simulink model "copy_final"  (R2013a)
settings: Solver=ode45  StartTime=0.0  StopTime=150  RelTol=1e-3
model workspace (MAT data in the model file):
  i = 2
undefined symbols (not defined in the file): sigbuilder_block
(part 1 of 3)
settings Model: Creator=User  LastModifiedBy=User
settings DebuggingCC: SolverPrmCheckMsg=none

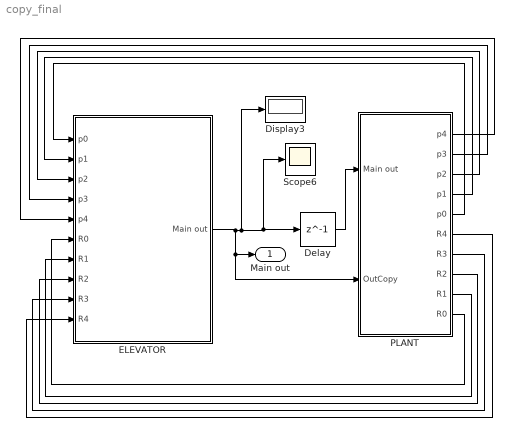
== system copy_final ==
  Delay : Delay  DelayLength=1  InitialCondition=0  SampleTime=1
  Display3 : Display
  ELEVATOR : Subsystem
  PLANT : Subsystem
  Scope6 : Scope
  Main out : Outport  OutDataTypeStr=int32
  wires:
  ELEVATOR/1(Main out) -> Scope6/1, Delay/1, Display3/1, PLANT/2(OutCopy), Main out/1
  Delay/1 -> PLANT/1(Main out)
  PLANT/5(p0) -> ELEVATOR/1(p0)
  PLANT/4("p1 ") -> ELEVATOR/2(p1)
  PLANT/3("p2 ") -> ELEVATOR/3(p2)
  PLANT/2("p3 ") -> ELEVATOR/4(p3)
  PLANT/1("p4 ") -> ELEVATOR/5(p4)
  PLANT/10(R0) -> ELEVATOR/6(R0)
  PLANT/9(R1) -> ELEVATOR/7(R1)
  PLANT/8(R2) -> ELEVATOR/8(R2)
  PLANT/7(R3) -> ELEVATOR/9(R3)
  PLANT/6(R4) -> ELEVATOR/10(R4)

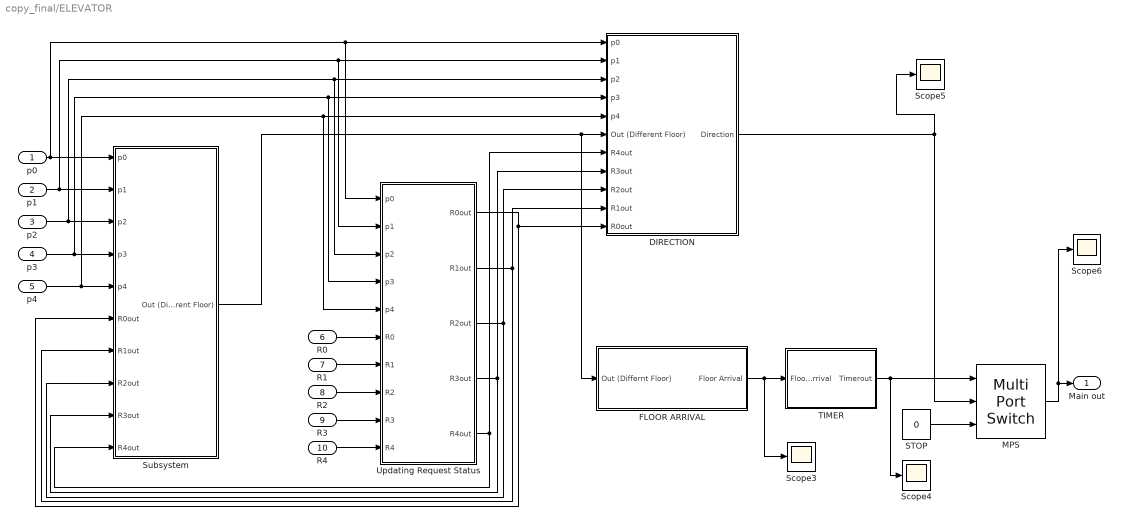
== system copy_final/ELEVATOR ==
  p0 : Inport  OutDataTypeStr=boolean
  p1 : Inport  Port=2  OutDataTypeStr=boolean
  p2 : Inport  Port=3  OutDataTypeStr=boolean
  p3 : Inport  Port=4  OutDataTypeStr=boolean
  p4 : Inport  Port=5  OutDataTypeStr=boolean  SampleTime=1
  R0 : Inport  Port=6  OutDataTypeStr=boolean
  R1 : Inport  Port=7  OutDataTypeStr=boolean
  R2 : Inport  Port=8  OutDataTypeStr=boolean
  R3 : Inport  Port=9  OutDataTypeStr=boolean
  R4 : Inport  Port=10  OutDataTypeStr=boolean
  DIRECTION : Subsystem
  FLOOR ARRIVAL : Subsystem
  "MPS " : MultiPortSwitch  DataPortOrder=Zero-based contiguous  Inputs=2  DiagnosticForDefault=None  OutDataTypeStr=int32  InputSameDT=on
  STOP : Constant  Value=0  OutDataTypeStr=int32
  Scope{3..6} (4 alike) : Scope
      Scope3 settings: SaveName=ScopeData76
      Scope4 settings: SaveName=ScopeData78
      Scope5 settings: SaveName=ScopeData8
      Scope6 settings: SaveName=ScopeData73
  Subsystem : Subsystem
  TIMER : Subsystem
  Updating Request Status : Subsystem
  Main out : Outport  OutDataTypeStr=int32
  wires:
  "MPS "/1 -> Scope6/1, Main out/1
  DIRECTION/1(" Direction ") -> "MPS "/2, Scope5/1
  TIMER/1(Timerout) -> "MPS "/1, Scope4/1
  FLOOR ARRIVAL/1(Floor Arrival) -> TIMER/1(Floor Arrival), Scope3/1
  p1/1 -> Updating Request Status/2(p1), DIRECTION/2(p1), Subsystem/2(p1)
  p2/1 -> Updating Request Status/3(p2), DIRECTION/3(p2), Subsystem/3(p2)
  p3/1 -> Updating Request Status/4(p3), DIRECTION/4(p3), Subsystem/4(p3)
  p4/1 -> Updating Request Status/5(p4), DIRECTION/5(p4), Subsystem/5(p4)
  Subsystem/1(Out (Different Floor)) -> FLOOR ARRIVAL/1(Out (Differnt Floor)), DIRECTION/6(Out (Different Floor))
  STOP/1 -> "MPS "/3
  Updating Request Status/1(R0out) -> Subsystem/6(R0out), DIRECTION/11(R0out)
  Updating Request Status/2(R1out) -> Subsystem/7(R1out), DIRECTION/10(R1out)
  Updating Request Status/3(R2out) -> Subsystem/8(R2out), DIRECTION/9(R2out)
  Updating Request Status/4(R3out) -> Subsystem/9(R3out), DIRECTION/8(R3out)
  Updating Request Status/5(R4out) -> Subsystem/10(R4out), DIRECTION/7(R4out)
  R1/1 -> Updating Request Status/7(R1)
  R2/1 -> Updating Request Status/8(R2)
  R3/1 -> Updating Request Status/9(R3)
  R4/1 -> Updating Request Status/10(R4)
  R0/1 -> Updating Request Status/6(R0)
  p0/1 -> DIRECTION/1(p0), Updating Request Status/1(p0), Subsystem/1(p0)

== system copy_final/PLANT ==
  Main out : Inport  OutDataTypeStr=int32
  OutCopy : Inport  Port=2  OutDataTypeStr=int32
  Calculating Position : Subsystem
  Live Request : Subsystem
  Position Id : Subsystem
  "p4 " : Outport  OutDataTypeStr=boolean
  "p3 " : Outport  Port=2  OutDataTypeStr=boolean
  "p2 " : Outport  Port=3  OutDataTypeStr=boolean
  "p1 " : Outport  Port=4  OutDataTypeStr=boolean
  p0 : Outport  Port=5  OutDataTypeStr=boolean
  R4 : Outport  Port=6  OutDataTypeStr=boolean
  R3 : Outport  Port=7  OutDataTypeStr=boolean
  R2 : Outport  Port=8  OutDataTypeStr=boolean
  R1 : Outport  Port=9  OutDataTypeStr=boolean
  R0 : Outport  Port=10  OutDataTypeStr=boolean
  wires:
  Live Request/1(R4) -> R4/1
  Live Request/2(R3) -> R3/1
  Live Request/3(R2) -> R2/1
  Live Request/4(R1) -> R1/1
  Live Request/5(R0) -> R0/1
  Position Id/1("p4 ") -> "p4 "/1
  Position Id/2("p3 ") -> "p3 "/1
  Position Id/3("p2 ") -> "p2 "/1
  Position Id/4("p1 ") -> "p1 "/1
  Position Id/5(p0) -> p0/1
  Calculating Position/1(position) -> Position Id/1(position)
  Main out/1 -> Calculating Position/1(Main out)
  OutCopy/1 -> Live Request/1(OutCopy)

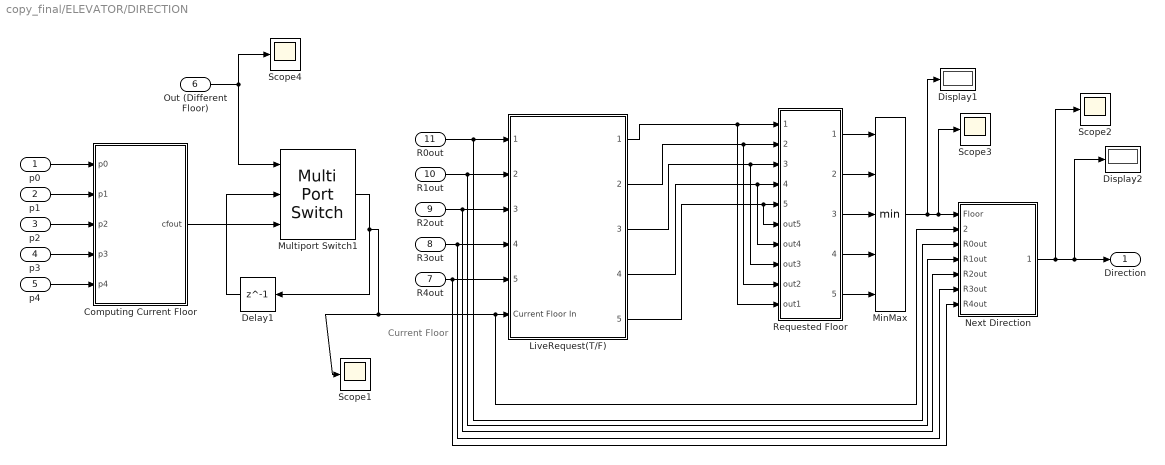
== system copy_final/ELEVATOR/DIRECTION ==
  note: Current Floor
  p0 : Inport  OutDataTypeStr=boolean
  p1 : Inport  Port=2  OutDataTypeStr=boolean
  p2 : Inport  Port=3  OutDataTypeStr=boolean
  p3 : Inport  Port=4  OutDataTypeStr=boolean
  p4 : Inport  Port=5  OutDataTypeStr=boolean
  Out (Different Floor) : Inport  Port=6  OutDataTypeStr=boolean
  R4out : Inport  Port=7  OutDataTypeStr=boolean
  R3out : Inport  Port=8  OutDataTypeStr=boolean
  R2out : Inport  Port=9  OutDataTypeStr=boolean
  R1out : Inport  Port=10  OutDataTypeStr=boolean
  R0out : Inport  Port=11  OutDataTypeStr=boolean
  "Computing Current Floor " : Subsystem
  Delay1 : Delay  DelayLength=1  SampleTime=1
  Display1 : Display
  Display2 : Display
  LiveRequest(T/F) : Subsystem
  MinMax : MinMax  Inputs=5  OutDataTypeStr=int32
  Multiport Switch1 : MultiPortSwitch  DataPortOrder=Zero-based contiguous  Inputs=2  DiagnosticForDefault=None  OutDataTypeStr=int32  InputSameDT=on
  Next Direction : Subsystem
  Requested Floor : Subsystem
  Scope{1..4} (4 alike) : Scope
      Scope1 settings: SaveName=ScopeData83
      Scope2 settings: SaveName=ScopeData47
      Scope3 settings: SaveName=ScopeData53
      Scope4 settings: SaveName=ScopeData84
  " Direction " : Outport  OutDataTypeStr=int32
  wires:
  p2/1 -> "Computing Current Floor "/3(p2)
  p3/1 -> "Computing Current Floor "/4(p3)
  p4/1 -> "Computing Current Floor "/5(p4)
  LiveRequest(T/F)/5 -> Requested Floor/6(out5), Requested Floor/5
  LiveRequest(T/F)/4 -> Requested Floor/4, Requested Floor/7(out4)
  Requested Floor/1(F0Out) -> MinMax/1
  Requested Floor/2(F1Out) -> MinMax/2
  Requested Floor/3(F2Out) -> MinMax/3
  Requested Floor/4(F3Out) -> MinMax/4
  Requested Floor/5(F4Out) -> MinMax/5
  p0/1 -> "Computing Current Floor "/1(p0)
  LiveRequest(T/F)/3 -> Requested Floor/8(out3), Requested Floor/3
  LiveRequest(T/F)/2 -> Requested Floor/9(out2), Requested Floor/2
  LiveRequest(T/F)/1 -> Requested Floor/10(out1), Requested Floor/1
  Next Direction/1(Direction) -> Scope2/1, Display2/1, " Direction "/1
  Multiport Switch1/1 -> Next Direction/2(Current Floor), LiveRequest(T/F)/6(Current Floor In), Scope1/1, Delay1/1
  MinMax/1 -> Next Direction/1(Floor), Scope3/1, Display1/1
  Out (Different Floor)/1 -> Scope4/1, Multiport Switch1/1
  p1/1 -> "Computing Current Floor "/2(p1)
  "Computing Current Floor "/1(cfout) -> Multiport Switch1/3
  Delay1/1 -> Multiport Switch1/2
  R1out/1 -> LiveRequest(T/F)/2, Next Direction/4(R1out)
  R2out/1 -> LiveRequest(T/F)/3, Next Direction/5(R2out)
  R3out/1 -> LiveRequest(T/F)/4, Next Direction/6(R3out)
  R4out/1 -> LiveRequest(T/F)/5, Next Direction/7(R4out)
  R0out/1 -> LiveRequest(T/F)/1, Next Direction/3(R0out)

== system copy_final/ELEVATOR/FLOOR ARRIVAL ==
  Out (Differnt Floor) : Inport  OutDataTypeStr=boolean
  " 1" : Logic  Operator=NOT  AllPortsSameDT=off  OutDataTypeStr=boolean
  Delay1 : Delay  DelayLength=1  SampleTime=1
  "Relational Operator " : Logic  AllPortsSameDT=off  OutDataTypeStr=boolean
  Scope{1..4} (4 alike) : Scope
      Scope1 settings: SaveName=ScopeData31
      Scope2 settings: SaveName=ScopeData32
      Scope3 settings: SaveName=ScopeData75
      Scope4 settings: SaveName=ScopeData77
  Floor Arrival : Outport  OutDataTypeStr=boolean
  wires:
  Out (Differnt Floor)/1 -> Scope1/1, Delay1/1, "Relational Operator "/1
  Delay1/1 -> Scope3/1, " 1"/1
  "Relational Operator "/1 -> Floor Arrival/1, Scope2/1
  " 1"/1 -> "Relational Operator "/2, Scope4/1

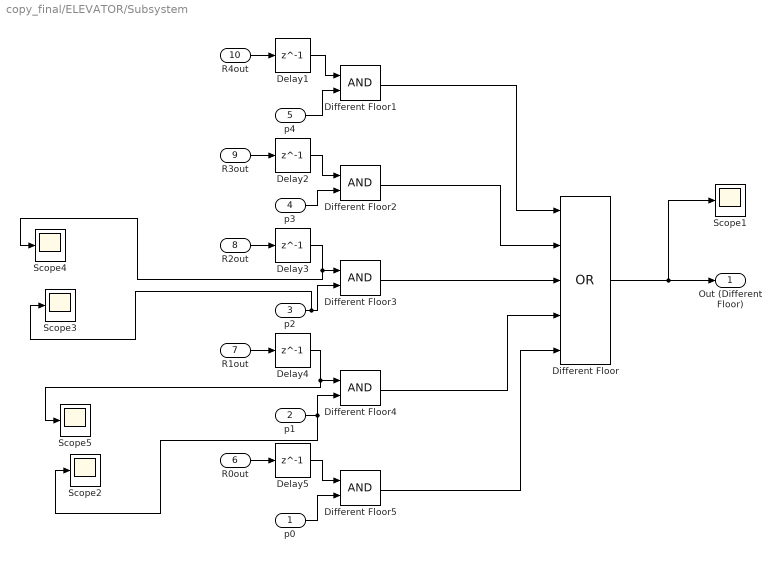
== system copy_final/ELEVATOR/Subsystem ==
  p0 : Inport  OutDataTypeStr=boolean
  p1 : Inport  Port=2  OutDataTypeStr=boolean
  p2 : Inport  Port=3  OutDataTypeStr=boolean
  p3 : Inport  Port=4  OutDataTypeStr=boolean
  p4 : Inport  Port=5  OutDataTypeStr=boolean  SampleTime=1
  R0out : Inport  Port=6  OutDataTypeStr=boolean
  R1out : Inport  Port=7  OutDataTypeStr=boolean
  R2out : Inport  Port=8  OutDataTypeStr=boolean
  R3out : Inport  Port=9  OutDataTypeStr=boolean
  R4out : Inport  Port=10  OutDataTypeStr=boolean
  Delay{1..5} (5 alike) : Delay  DelayLength=1  SampleTime=1
  Different Floor : Logic  Operator=OR  Inputs=5  AllPortsSameDT=off  OutDataTypeStr=boolean
  Different Floor{1..5} (5 alike) : Logic  AllPortsSameDT=off  OutDataTypeStr=boolean
  Scope{1..5} (5 alike) : Scope
      Scope1 settings: SaveName=ScopeData45
      Scope2 settings: SaveName=ScopeData46
      Scope3 settings: SaveName=ScopeData65
      Scope4 settings: SaveName=ScopeData66
      Scope5 settings: SaveName=ScopeData44
  Out (Different Floor) : Outport  OutDataTypeStr=boolean
  wires:
  R4out/1 -> Delay1/1
  p4/1 -> Different Floor1/2
  R3out/1 -> Delay2/1
  p3/1 -> Different Floor2/2
  R2out/1 -> Delay3/1
  p2/1 -> Scope3/1, Different Floor3/2
  R1out/1 -> Delay4/1
  p1/1 -> Scope2/1, Different Floor4/2
  R0out/1 -> Delay5/1
  p0/1 -> Different Floor5/2
  Different Floor1/1 -> Different Floor/1
  Different Floor2/1 -> Different Floor/2
  Different Floor3/1 -> Different Floor/3
  Different Floor4/1 -> Different Floor/4
  Different Floor5/1 -> Different Floor/5
  Different Floor/1 -> Scope1/1, Out (Different Floor)/1
  Delay1/1 -> Different Floor1/1
  Delay2/1 -> Different Floor2/1
  Delay3/1 -> Different Floor3/1, Scope4/1
  Delay4/1 -> Scope5/1, Different Floor4/1
  Delay5/1 -> Different Floor5/1

== system copy_final/ELEVATOR/TIMER ==
  Floor Arrival : Inport  OutDataTypeStr=boolean
  Delay1 : Delay  DelayLength=10  SampleTime=1
  Logical Operator1 : Logic  Operator=OR  AllPortsSameDT=off  OutDataTypeStr=boolean
  Scope{1..4} (4 alike) : Scope
      Scope1 settings: SaveName=ScopeData33
      Scope2 settings: SaveName=ScopeData30
      Scope3 settings: SaveName=ScopeData48
      Scope4 settings: SaveName=ScopeData50
  Toggle1 : Subsystem
  Timerout : Outport  OutDataTypeStr=boolean
  wires:
  Toggle1/1(Timerout) -> Timerout/1, Scope4/1
  Logical Operator1/1 -> Scope3/1, Toggle1/1(Toggle In)
  Floor Arrival/1 -> Scope2/1, Logical Operator1/2, Delay1/1
  Delay1/1 -> Scope1/1, Logical Operator1/1

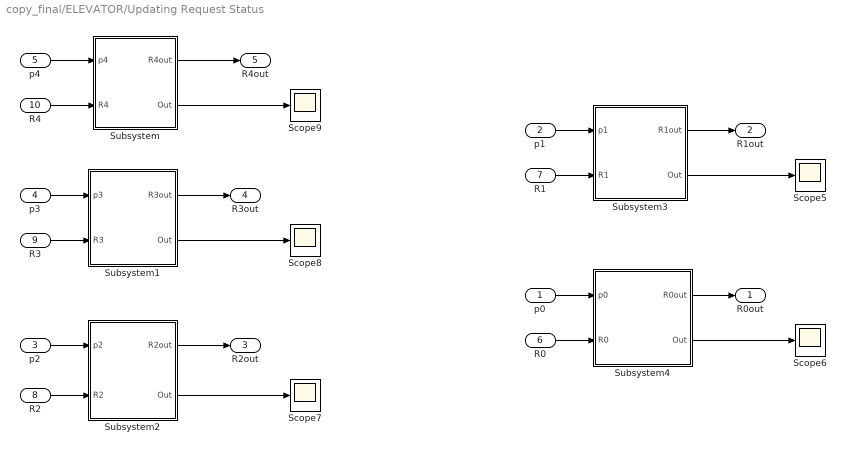
== system copy_final/ELEVATOR/Updating Request Status ==
  p0 : Inport
  p1 : Inport  Port=2  OutDataTypeStr=boolean
  p2 : Inport  Port=3  OutDataTypeStr=boolean
  p3 : Inport  Port=4  OutDataTypeStr=boolean
  p4 : Inport  Port=5  OutDataTypeStr=boolean
  R0 : Inport  Port=6
  R1 : Inport  Port=7  OutDataTypeStr=boolean
  R2 : Inport  Port=8  OutDataTypeStr=boolean
  R3 : Inport  Port=9  OutDataTypeStr=boolean
  R4 : Inport  Port=10  OutDataTypeStr=boolean
  Scope{5..9} (5 alike) : Scope
      Scope5 settings: SaveName=ScopeData14
      Scope6 settings: SaveName=ScopeData15
      Scope7 settings: SaveName=ScopeData16
      Scope8 settings: SaveName=ScopeData17
      Scope9 settings: SaveName=ScopeData18
  Subsystem : Subsystem
  Subsystem1 : Subsystem
  Subsystem2 : Subsystem
  Subsystem3 : Subsystem
  Subsystem4 : Subsystem
  R0out : Outport  OutDataTypeStr=boolean
  R1out : Outport  Port=2  OutDataTypeStr=boolean
  R2out : Outport  Port=3  OutDataTypeStr=boolean
  R3out : Outport  Port=4  OutDataTypeStr=boolean
  R4out : Outport  Port=5  OutDataTypeStr=boolean
  wires:
  p4/1 -> Subsystem/1(p4)
  R4/1 -> Subsystem/2(R4)
  Subsystem/1(R4out) -> R4out/1
  p3/1 -> Subsystem1/1(p3)
  R3/1 -> Subsystem1/2(R3)
  Subsystem1/1(R3out) -> R3out/1
  p2/1 -> Subsystem2/1(p2)
  R2/1 -> Subsystem2/2(R2)
  p0/1 -> Subsystem4/1(p0)
  R0/1 -> Subsystem4/2(R0)
  Subsystem4/1(R0out) -> R0out/1
  Subsystem/2(Out) -> Scope9/1
  Subsystem1/2(Out) -> Scope8/1
  Subsystem2/1(R2out) -> R2out/1
  Subsystem2/2(Out) -> Scope7/1
  Subsystem4/2(Out) -> Scope6/1
  p1/1 -> Subsystem3/1(p1)
  R1/1 -> Subsystem3/2(R1)
  Subsystem3/1(R1out) -> R1out/1
  Subsystem3/2(Out) -> Scope5/1

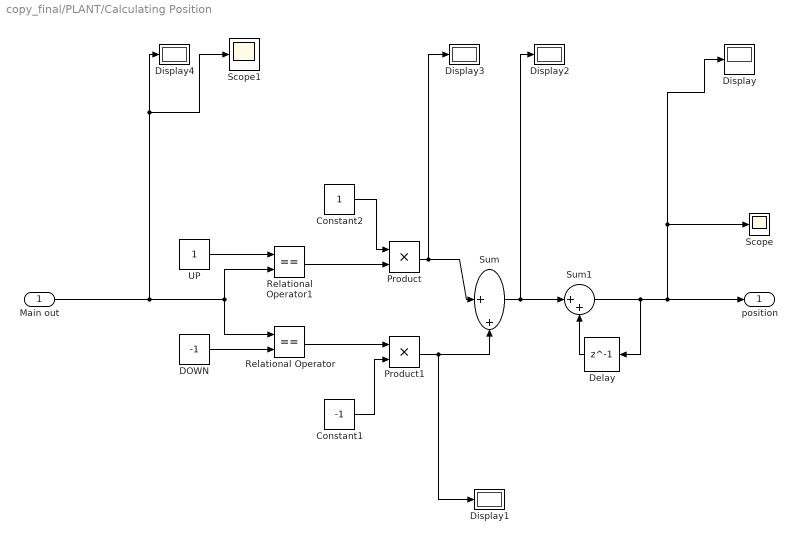
== system copy_final/PLANT/Calculating Position ==
  Main out : Inport  OutDataTypeStr=int32
  Constant1 : Constant  Value=-1  OutDataTypeStr=int32
  Constant2 : Constant  OutDataTypeStr=int32
  DOWN : Constant  Value=-1  OutDataTypeStr=int32
  Delay : Delay  DelayLength=1  InitialCondition=0  SampleTime=1
  Display{,1..4} (5 alike) : Display
  Product : Product  OutDataTypeStr=int32
  Product1 : Product  OutDataTypeStr=int32
  Relational Operator : RelationalOperator  Operator===  OutDataTypeStr=boolean
  Relational Operator1 : RelationalOperator  Operator===  OutDataTypeStr=boolean
  Scope : Scope
      settings: SaveName=ScopeData74
  Scope1 : Scope
      settings: SaveName=ScopeData63
  Sum : Sum  Inputs=|++  AccumDataTypeStr=int32  OutDataTypeStr=int32
  Sum1 : Sum  Inputs=|++  AccumDataTypeStr=int32  OutDataTypeStr=int32
  UP : Constant  OutDataTypeStr=int32
  position : Outport  OutDataTypeStr=int32
  wires:
  DOWN/1 -> Relational Operator/2
  UP/1 -> Relational Operator1/1
  Relational Operator1/1 -> Product/2
  Constant2/1 -> Product/1
  Relational Operator/1 -> Product1/1
  Constant1/1 -> Product1/2
  Product/1 -> Sum/1, Display3/1
  Product1/1 -> Sum/2, Display1/1
  Sum/1 -> Sum1/1, Display2/1
  Main out/1 -> Relational Operator/1, Relational Operator1/2, Scope1/1, Display4/1
  Sum1/1 -> Delay/1, Display/1, Scope/1, position/1
  Delay/1 -> Sum1/2

== system copy_final/PLANT/Live Request ==
  OutCopy : Inport  OutDataTypeStr=int32
  Demux : Demux  Outputs=5
  Different TestCases : Subsystem
  Scope{1..3,6..8} (6 alike) : Scope
      Scope2 settings: TimeRange=50  SaveName=ScopeData2
      Scope3 settings: SaveName=ScopeData91
      Scope6 settings: SaveName=ScopeData3
      Scope7 settings: SaveName=ScopeData4
      Scope8 settings: SaveName=ScopeData5
  R4 : Outport  OutDataTypeStr=boolean
  R3 : Outport  Port=2  OutDataTypeStr=boolean
  R2 : Outport  Port=3  OutDataTypeStr=boolean
  R1 : Outport  Port=4  OutDataTypeStr=boolean
  R0 : Outport  Port=5  OutDataTypeStr=boolean
  wires:
  Demux/1 -> Scope2/1, R4/1
  Demux/2 -> R3/1, Scope1/1
  Demux/4 -> Scope7/1, R1/1
  Demux/5 -> Scope8/1, R0/1
  Demux/3 -> Scope6/1, R2/1
  OutCopy/1 -> Scope3/1
  Different TestCases/15(TestCase15) -> Demux/1

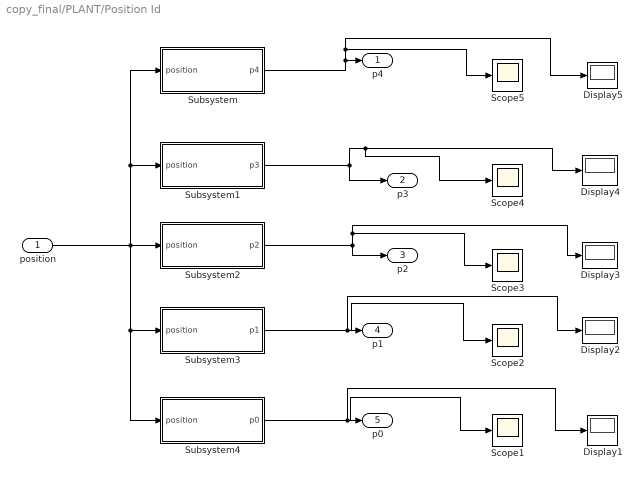
== system copy_final/PLANT/Position Id ==
  position : Inport  OutDataTypeStr=int32
  Display{1..5} (5 alike) : Display
  Scope{1..5} (5 alike) : Scope
      Scope1 settings: SaveName=ScopeData7
      Scope2 settings: SaveName=ScopeData40
      Scope3 settings: SaveName=ScopeData41
      Scope4 settings: SaveName=ScopeData42
      Scope5 settings: SaveName=ScopeData43
  Subsystem : Subsystem
  Subsystem1 : Subsystem
  Subsystem2 : Subsystem
  Subsystem3 : Subsystem
  Subsystem4 : Subsystem
  "p4 " : Outport  OutDataTypeStr=boolean
  "p3 " : Outport  Port=2  OutDataTypeStr=boolean
  "p2 " : Outport  Port=3  OutDataTypeStr=boolean
  "p1 " : Outport  Port=4  OutDataTypeStr=boolean
  p0 : Outport  Port=5  OutDataTypeStr=boolean
  wires:
  position/1 -> Subsystem4/1(position), Subsystem3/1(position), Subsystem2/1(position), Subsystem/1(position), Subsystem1/1(position)
  Subsystem/1("p4 ") -> Display5/1, Scope5/1, "p4 "/1
  Subsystem1/1("p3 ") -> Scope4/1, Display4/1, "p3 "/1
  Subsystem2/1("p2 ") -> Scope3/1, Display3/1, "p2 "/1
  Subsystem3/1("p1 ") -> Display2/1, Scope2/1, "p1 "/1
  Subsystem4/1("p0 ") -> Display1/1, Scope1/1, p0/1

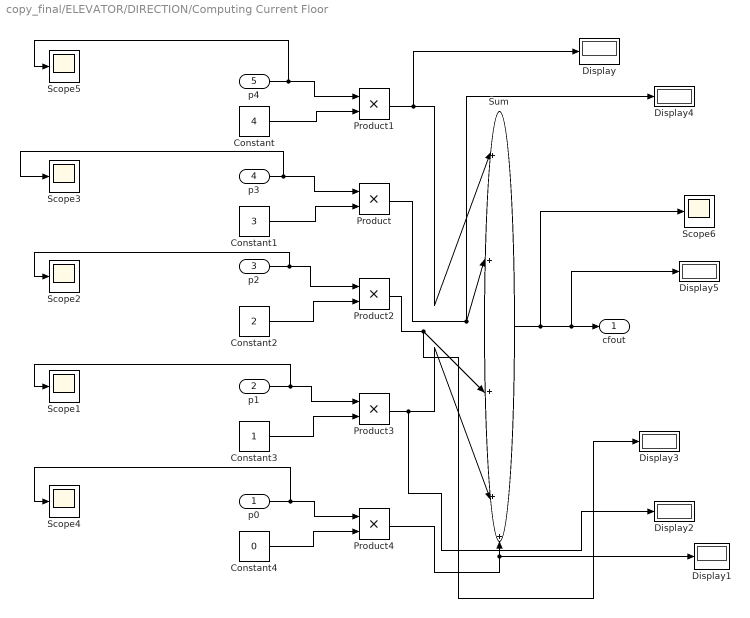
== system copy_final/ELEVATOR/DIRECTION/Computing Current Floor  ==
  p0 : Inport  OutDataTypeStr=boolean
  p1 : Inport  Port=2  OutDataTypeStr=boolean
  p2 : Inport  Port=3  OutDataTypeStr=boolean
  p3 : Inport  Port=4  OutDataTypeStr=boolean
  p4 : Inport  Port=5  OutDataTypeStr=boolean
  Constant : Constant  Value=4  OutDataTypeStr=int32
  Constant1 : Constant  Value=3  OutDataTypeStr=int32
  Constant2 : Constant  Value=2  OutDataTypeStr=int32
  Constant3 : Constant  OutDataTypeStr=int32
  Constant4 : Constant  Value=0  OutDataTypeStr=int32
  Display{,1..5} (6 alike) : Display
  Product{,1..4} (5 alike) : Product  OutDataTypeStr=int32
  Scope{1..6} (6 alike) : Scope
      Scope1 settings: SaveName=ScopeData58
      Scope2 settings: SaveName=ScopeData59
      Scope3 settings: SaveName=ScopeData60
      Scope4 settings: SaveName=ScopeData57
      Scope5 settings: SaveName=ScopeData61
      Scope6 settings: SaveName=ScopeData62
  Sum : Sum  Inputs=|+++++  AccumDataTypeStr=int32  OutDataTypeStr=int32
  cfout : Outport  OutDataTypeStr=int32
  wires:
  p4/1 -> Scope5/1, Product1/1
  Constant/1 -> Product1/2
  p3/1 -> Product/1, Scope3/1
  Constant1/1 -> Product/2
  p2/1 -> Scope2/1, Product2/1
  Constant2/1 -> Product2/2
  p1/1 -> Scope1/1, Product3/1
  Constant3/1 -> Product3/2
  p0/1 -> Scope4/1, Product4/1
  Constant4/1 -> Product4/2
  Product1/1 -> Display/1, Sum/1
  Product4/1 -> Sum/5, Display1/1
  Product/1 -> Sum/2, Display4/1
  Product2/1 -> Display3/1, Sum/3
  Product3/1 -> Display2/1, Sum/4
  Sum/1 -> Scope6/1, Display5/1, cfout/1

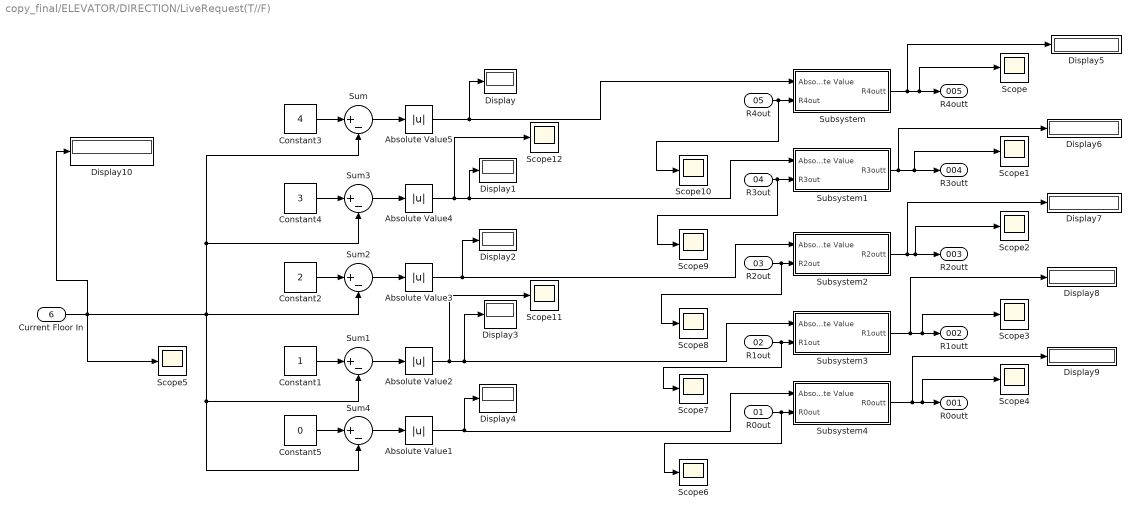
== system copy_final/ELEVATOR/DIRECTION/LiveRequest(T//F) ==
  R0out : Inport  Port=01  OutDataTypeStr=boolean
  R1out : Inport  Port=02  OutDataTypeStr=boolean
  R2out : Inport  Port=03  OutDataTypeStr=boolean
  R3out : Inport  Port=04  OutDataTypeStr=boolean
  R4out : Inport  Port=05  OutDataTypeStr=boolean
  Current Floor In : Inport  Port=6  OutDataTypeStr=int32
  Absolute Value{1..5} (5 alike) : Abs  OutDataTypeStr=int32
  Constant1 : Constant  OutDataTypeStr=int32
  Constant2 : Constant  Value=2  OutDataTypeStr=int32
  Constant3 : Constant  Value=4  OutDataTypeStr=int32
  Constant4 : Constant  Value=3  OutDataTypeStr=int32
  Constant5 : Constant  Value=0  OutDataTypeStr=int32
  Display{,1..10} (11 alike) : Display
  Scope{,1..12} (13 alike) : Scope
      Scope settings: SaveName=ScopeData35
      Scope1 settings: SaveName=ScopeData36
      Scope10 settings: SaveName=ScopeData71
      Scope11 settings: SaveName=ScopeData51
      Scope12 settings: SaveName=ScopeData52
      Scope2 settings: SaveName=ScopeData37
      Scope3 settings: SaveName=ScopeData38
      Scope4 settings: SaveName=ScopeData39
      Scope5 settings: SaveName=ScopeData64
      Scope6 settings: SaveName=ScopeData67
      Scope7 settings: SaveName=ScopeData68
      Scope8 settings: SaveName=ScopeData69
      Scope9 settings: SaveName=ScopeData70
  Subsystem : Subsystem
  Subsystem1 : Subsystem
  Subsystem2 : Subsystem
  Subsystem3 : Subsystem
  Subsystem4 : Subsystem
  Sum{,1..2,4} (4 alike) : Sum  Inputs=|+-  AccumDataTypeStr=int32
  Sum3 : Sum  Inputs=|+-  OutDataTypeStr=int32
  R0outt : Outport  Port=001  OutDataTypeStr=int32
  R1outt : Outport  Port=002  OutDataTypeStr=int32
  R2outt : Outport  Port=003  OutDataTypeStr=int32
  R3outt : Outport  Port=004  OutDataTypeStr=int32
  R4outt : Outport  Port=005  OutDataTypeStr=int32
  wires:
  Subsystem/1(R4outt) -> Display5/1, Scope/1, R4outt/1
  R4out/1 -> Scope10/1, Subsystem/2(R4out)
  Subsystem1/1(R3outt) -> Display6/1, Scope1/1, R3outt/1
  R3out/1 -> Scope9/1, Subsystem1/2(R3out)
  Subsystem2/1(R2outt) -> Display7/1, Scope2/1, R2outt/1
  R2out/1 -> Scope8/1, Subsystem2/2(R2out)
  R1out/1 -> Scope7/1, Subsystem3/2(R1out)
  Subsystem4/1(R0outt) -> Display9/1, Scope4/1, R0outt/1
  R0out/1 -> Scope6/1, Subsystem4/2(R0out)
  Sum/1 -> Absolute Value5/1
  Constant3/1 -> Sum/1
  Absolute Value5/1 -> Subsystem/1(Absolute Value), Display/1
  Constant4/1 -> Sum3/1
  Sum3/1 -> Absolute Value4/1
  Sum2/1 -> Absolute Value3/1
  Constant2/1 -> Sum2/1
  Absolute Value3/1 -> Display2/1, Subsystem2/1(Absolute Value)
  Constant1/1 -> Sum1/1
  Sum1/1 -> Absolute Value2/1
  Sum4/1 -> Absolute Value1/1
  Constant5/1 -> Sum4/1
  Absolute Value1/1 -> Subsystem4/1(Absolute Value), Display4/1
  Subsystem3/1(R1outt) -> Display8/1, Scope3/1, R1outt/1
  Absolute Value2/1 -> Subsystem3/1(Absolute Value), Display3/1, Scope11/1
  Absolute Value4/1 -> Scope12/1, Subsystem1/1(Absolute Value), Display1/1
  Current Floor In/1 -> Sum4/2, Sum1/2, Sum3/2, Sum/2, Sum2/2, Display10/1, Scope5/1

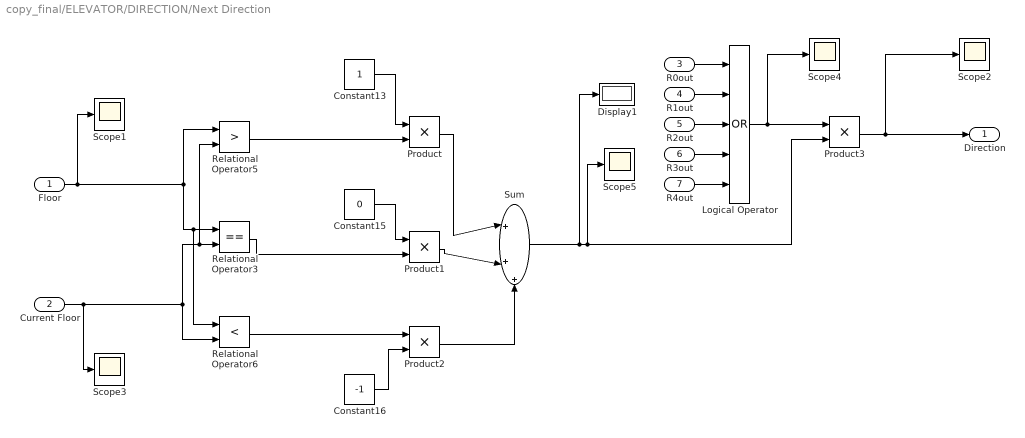
== system copy_final/ELEVATOR/DIRECTION/Next Direction ==
  Floor : Inport  OutDataTypeStr=int32
  Current Floor : Inport  Port=2  OutDataTypeStr=int32
  R0out : Inport  Port=3  OutDataTypeStr=boolean
  R1out : Inport  Port=4  OutDataTypeStr=boolean
  R2out : Inport  Port=5  OutDataTypeStr=boolean
  R3out : Inport  Port=6  OutDataTypeStr=boolean
  R4out : Inport  Port=7  OutDataTypeStr=boolean
  Constant13 : Constant  OutDataTypeStr=int32
  Constant15 : Constant  Value=0  OutDataTypeStr=int32
  Constant16 : Constant  Value=-1  OutDataTypeStr=int32
  Display1 : Display
  Logical Operator : Logic  Operator=OR  Inputs=5  AllPortsSameDT=off  OutDataTypeStr=boolean
  Product{,1..3} (4 alike) : Product  OutDataTypeStr=int32
  Relational Operator3 : RelationalOperator  Operator===  OutDataTypeStr=boolean
  Relational Operator5 : RelationalOperator  Operator=>  OutDataTypeStr=boolean
  Relational Operator6 : RelationalOperator  Operator=<  OutDataTypeStr=boolean
  Scope{1..5} (5 alike) : Scope
      Scope1 settings: SaveName=ScopeData29
      Scope2 settings: SaveName=ScopeData54
      Scope3 settings: SaveName=ScopeData56
      Scope4 settings: SaveName=ScopeData89
      Scope5 settings: SaveName=ScopeData90
  Sum : Sum  Inputs=|+++  AccumDataTypeStr=int32  OutDataTypeStr=int32
  Direction : Outport  OutDataTypeStr=int32
  wires:
  Constant16/1 -> Product2/2
  Relational Operator6/1 -> Product2/1
  Floor/1 -> Relational Operator6/1, Relational Operator3/1, Relational Operator5/1, Scope1/1
  Sum/1 -> Product3/2, Scope5/1, Display1/1
  Constant15/1 -> Product1/1
  Current Floor/1 -> Relational Operator5/2, Relational Operator3/2, Relational Operator6/2, Scope3/1
  Product2/1 -> Sum/3
  Relational Operator3/1 -> Product1/2
  Relational Operator5/1 -> Product/2
  Product/1 -> Sum/1
  Constant13/1 -> Product/1
  Product1/1 -> Sum/2
  R1out/1 -> Logical Operator/2
  R2out/1 -> Logical Operator/3
  R3out/1 -> Logical Operator/4
  R4out/1 -> Logical Operator/5
  R0out/1 -> Logical Operator/1
  Logical Operator/1 -> Scope4/1, Product3/1
  Product3/1 -> Scope2/1, Direction/1

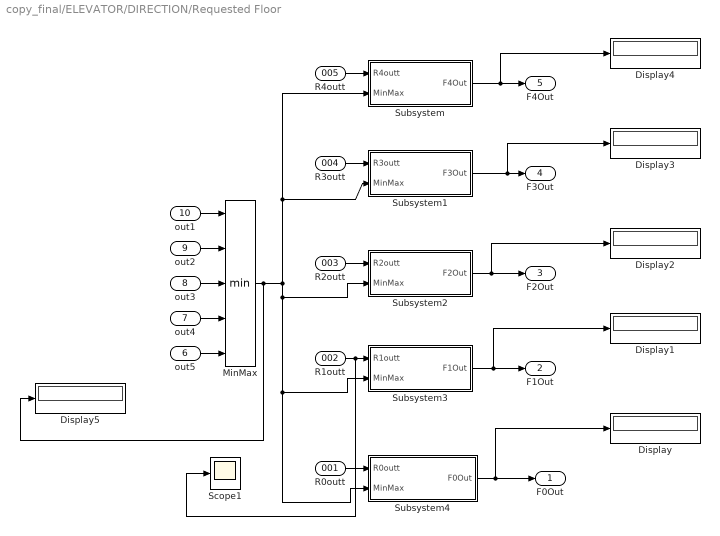
== system copy_final/ELEVATOR/DIRECTION/Requested Floor ==
  R0outt : Inport  Port=001  OutDataTypeStr=int32
  R1outt : Inport  Port=002  OutDataTypeStr=int32
  R2outt : Inport  Port=003  OutDataTypeStr=int32
  R3outt : Inport  Port=004  OutDataTypeStr=int32
  R4outt : Inport  Port=005  OutDataTypeStr=int32
  out5 : Inport  Port=6  OutDataTypeStr=int32
  out4 : Inport  Port=7  OutDataTypeStr=int32
  out3 : Inport  Port=8  OutDataTypeStr=int32
  out2 : Inport  Port=9  OutDataTypeStr=int32
  out1 : Inport  Port=10  OutDataTypeStr=int32
  Display{,1..5} (6 alike) : Display
  MinMax : MinMax  Inputs=5  OutDataTypeStr=int32
  Scope1 : Scope
      settings: SaveName=ScopeData72
  Subsystem : Subsystem
  Subsystem1 : Subsystem
  Subsystem2 : Subsystem
  Subsystem3 : Subsystem
  Subsystem4 : Subsystem
  F0Out : Outport  OutDataTypeStr=int32
  F1Out : Outport  Port=2  OutDataTypeStr=int32
  F2Out : Outport  Port=3  OutDataTypeStr=int32
  F3Out : Outport  Port=4  OutDataTypeStr=int32
  F4Out : Outport  Port=5  OutDataTypeStr=int32
  wires:
  out1/1 -> MinMax/1
  out2/1 -> MinMax/2
  out3/1 -> MinMax/3
  out4/1 -> MinMax/4
  out5/1 -> MinMax/5
  R4outt/1 -> Subsystem/1(R4outt)
  R3outt/1 -> Subsystem1/1(R3outt)
  R2outt/1 -> Subsystem2/1(R2outt)
  R1outt/1 -> Subsystem3/1(R1outt), Scope1/1
  R0outt/1 -> Subsystem4/1(R0outt)
  Subsystem/1(F4Out) -> Display4/1, F4Out/1
  Subsystem2/1(F2Out) -> Display2/1, F2Out/1
  Subsystem4/1(F0Out) -> Display/1, F0Out/1
  Subsystem3/1(F1Out) -> Display1/1, F1Out/1
  Subsystem1/1(F3Out) -> Display3/1, F3Out/1
  MinMax/1 -> Display5/1, Subsystem2/2(MinMax), Subsystem4/2(MinMax), Subsystem3/2(MinMax), Subsystem/2(MinMax), Subsystem1/2(MinMax)

== system copy_final/ELEVATOR/TIMER/Toggle1 ==
  Toggle In : Inport  OutDataTypeStr=boolean
  Data Type Conversion : DataTypeConversion  OutDataTypeStr=boolean
  Delay : Delay  DelayLength=1  InitialCondition=0  SampleTime=1
  Logical Operator2 : Logic  Operator=NOT  AllPortsSameDT=off  OutDataTypeStr=boolean
  "MPS " : MultiPortSwitch  DataPortOrder=Zero-based contiguous  Inputs=2  DiagnosticForDefault=None  OutDataTypeStr=int32
  Scope1 : Scope
      settings: SaveName=ScopeData49
  Scope2 : Scope
      settings: SaveName=ScopeData34
  Timerout : Outport  OutDataTypeStr=boolean
  wires:
  Toggle In/1 -> Scope1/1, "MPS "/1
  Delay/1 -> "MPS "/2, Logical Operator2/1
  "MPS "/1 -> Data Type Conversion/1
  Logical Operator2/1 -> "MPS "/3
  Data Type Conversion/1 -> Delay/1, Timerout/1, Scope2/1

== system copy_final/ELEVATOR/Updating Request Status/Subsystem ==
  p4 : Inport  OutDataTypeStr=boolean
  R4 : Inport  Port=2  OutDataTypeStr=boolean
  Delay : Delay  DelayLength=1  SampleTime=1
  Logical Operator1 : Logic  Operator=NOT  AllPortsSameDT=off  OutDataTypeStr=boolean
  Logical Operator2 : Logic  AllPortsSameDT=off  OutDataTypeStr=boolean
  Logical Operator3 : Logic  AllPortsSameDT=off  OutDataTypeStr=boolean
  MTP : MultiPortSwitch  DataPortOrder=Zero-based contiguous  Inputs=2  DiagnosticForDefault=None  OutDataTypeStr=int32
  Scope{1..4} (4 alike) : Scope
      Scope1 settings: SaveName=ScopeData24
      Scope2 settings: SaveName=ScopeData22
      Scope3 settings: SaveName=ScopeData13
      Scope4 settings: SaveName=ScopeData92
  TRUE : Constant  OutDataTypeStr=boolean
  R4out : Outport  OutDataTypeStr=boolean
  Out : Outport  Port=2  OutDataTypeStr=boolean
  wires:
  MTP/1 -> Logical Operator3/2
  Logical Operator2/1 -> Scope2/1, MTP/1
  Logical Operator1/1 -> Scope3/1, Logical Operator3/1, Logical Operator2/1
  Logical Operator3/1 -> Delay/1, Out/1, R4out/1
  p4/1 -> Logical Operator1/1
  R4/1 -> Scope1/1, Logical Operator2/2
  Delay/1 -> MTP/2
  TRUE/1 -> Scope4/1, MTP/3

== system copy_final/ELEVATOR/Updating Request Status/Subsystem1 ==
  p3 : Inport  OutDataTypeStr=boolean
  R3 : Inport  Port=2  OutDataTypeStr=boolean
  Delay : Delay  DelayLength=1  SampleTime=1
  Logical Operator1 : Logic  Operator=NOT  AllPortsSameDT=off  OutDataTypeStr=boolean
  Logical Operator2 : Logic  AllPortsSameDT=off  OutDataTypeStr=boolean
  Logical Operator3 : Logic  AllPortsSameDT=off  OutDataTypeStr=boolean
  MTP : MultiPortSwitch  DataPortOrder=Zero-based contiguous  Inputs=2  DiagnosticForDefault=None  OutDataTypeStr=int32
  Scope{1..5,7} (6 alike) : Scope
      Scope1 settings: SaveName=ScopeData12
      Scope2 settings: SaveName=ScopeData21
      Scope3 settings: SaveName=ScopeData25
      Scope4 settings: SaveName=ScopeData55
      Scope5 settings: SaveName=ScopeData94
      Scope7 settings: SaveName=ScopeData93
  TRUE : Constant  OutDataTypeStr=boolean
  R3out : Outport  OutDataTypeStr=boolean
  Out : Outport  Port=2  OutDataTypeStr=boolean
  wires:
  MTP/1 -> Logical Operator3/2
  Logical Operator2/1 -> Scope2/1, MTP/1
  Logical Operator1/1 -> Scope3/1, Logical Operator3/1, Logical Operator2/1
  Logical Operator3/1 -> Delay/1, Scope4/1, Out/1, R3out/1
  p3/1 -> Scope5/1, Logical Operator1/1
  R3/1 -> Scope1/1, Logical Operator2/2
  Delay/1 -> MTP/2
  TRUE/1 -> Scope7/1, MTP/3

== system copy_final/ELEVATOR/Updating Request Status/Subsystem2 ==
  p2 : Inport  OutDataTypeStr=boolean
  R2 : Inport  Port=2  OutDataTypeStr=boolean
  Delay : Delay  DelayLength=1  SampleTime=1
  Logical Operator1 : Logic  Operator=NOT  AllPortsSameDT=off  OutDataTypeStr=boolean
  Logical Operator2 : Logic  AllPortsSameDT=off  OutDataTypeStr=boolean
  Logical Operator3 : Logic  AllPortsSameDT=off  OutDataTypeStr=boolean
  MTP : MultiPortSwitch  DataPortOrder=Zero-based contiguous  Inputs=2  DiagnosticForDefault=None  OutDataTypeStr=int32
  Scope{1..7} (7 alike) : Scope
      Scope1 settings: SaveName=ScopeData11
      Scope2 settings: SaveName=ScopeData20
      Scope3 settings: SaveName=ScopeData26
      Scope4 settings: SaveName=ScopeData79
      Scope5 settings: SaveName=ScopeData85
      Scope6 settings: SaveName=ScopeData81
      Scope7 settings: SaveName=ScopeData87
  TRUE : Constant  OutDataTypeStr=boolean
  R2out : Outport  OutDataTypeStr=boolean
  Out : Outport  Port=2  OutDataTypeStr=boolean
  wires:
  MTP/1 -> Scope6/1, Logical Operator3/2
  Logical Operator2/1 -> Scope2/1, MTP/1
  Logical Operator1/1 -> Scope3/1, Logical Operator3/1, Logical Operator2/1
  Logical Operator3/1 -> Scope4/1, Out/1, R2out/1, Delay/1
  p2/1 -> Scope5/1, Logical Operator1/1
  R2/1 -> Scope1/1, Logical Operator2/2
  Delay/1 -> Scope7/1, MTP/2
  TRUE/1 -> MTP/3

== system copy_final/ELEVATOR/Updating Request Status/Subsystem3 ==
  p1 : Inport  OutDataTypeStr=boolean
  R1 : Inport  Port=2  OutDataTypeStr=boolean
  Delay : Delay  DelayLength=1  SampleTime=1
  Logical Operator1 : Logic  Operator=NOT  AllPortsSameDT=off  OutDataTypeStr=boolean
  Logical Operator2 : Logic  AllPortsSameDT=off  OutDataTypeStr=boolean
  Logical Operator3 : Logic  AllPortsSameDT=off  OutDataTypeStr=boolean
  MTP : MultiPortSwitch  DataPortOrder=Zero-based contiguous  Inputs=2  DiagnosticForDefault=None  OutDataTypeStr=int32
  Scope{1..7} (7 alike) : Scope
      Scope1 settings: SaveName=ScopeData6
      Scope2 settings: SaveName=ScopeData9
      Scope3 settings: SaveName=ScopeData19
      Scope4 settings: SaveName=ScopeData27
      Scope5 settings: SaveName=ScopeData80
      Scope6 settings: SaveName=ScopeData82
      Scope7 settings: SaveName=ScopeData86
  TRUE : Constant  OutDataTypeStr=boolean
  R1out : Outport  OutDataTypeStr=boolean
  Out : Outport  Port=2  OutDataTypeStr=boolean
  wires:
  MTP/1 -> Scope6/1, Logical Operator3/2
  Logical Operator2/1 -> Scope2/1, MTP/1
  Logical Operator1/1 -> Scope3/1, Logical Operator3/1, Logical Operator2/1
  Logical Operator3/1 -> Scope4/1, Out/1, R1out/1, Delay/1
  p1/1 -> Scope5/1, Logical Operator1/1
  R1/1 -> Scope1/1, Logical Operator2/2
  Delay/1 -> Scope7/1, MTP/2
  TRUE/1 -> MTP/3

== system copy_final/ELEVATOR/Updating Request Status/Subsystem4 ==
  p0 : Inport  OutDataTypeStr=boolean
  R0 : Inport  Port=2  OutDataTypeStr=boolean
  Delay : Delay  DelayLength=1  SampleTime=1
  Logical Operator1 : Logic  Operator=NOT  AllPortsSameDT=off  OutDataTypeStr=boolean
  Logical Operator2 : Logic  AllPortsSameDT=off  OutDataTypeStr=boolean
  Logical Operator3 : Logic  AllPortsSameDT=off  OutDataTypeStr=boolean
  MTP : MultiPortSwitch  DataPortOrder=Zero-based contiguous  Inputs=2  DiagnosticForDefault=None  OutDataTypeStr=int32
  Scope{1..4} (4 alike) : Scope
      Scope1 settings: SaveName=ScopeData10
      Scope2 settings: SaveName=ScopeData23
      Scope3 settings: SaveName=ScopeData28
      Scope4 settings: SaveName=ScopeData88
  TRUE : Constant  OutDataTypeStr=boolean
  R0out : Outport  OutDataTypeStr=boolean
  Out : Outport  Port=2  OutDataTypeStr=boolean
  wires:
  MTP/1 -> Logical Operator3/2
  Logical Operator2/1 -> Scope2/1, MTP/1
  Logical Operator1/1 -> Scope3/1, Logical Operator3/1, Logical Operator2/1
  Logical Operator3/1 -> Delay/1, Out/1, R0out/1
  p0/1 -> Logical Operator1/1
  R0/1 -> Scope1/1, Logical Operator2/2
  TRUE/1 -> MTP/3
  Delay/1 -> Scope4/1, MTP/2
